simulink model "p7_2"  (R2024b)
settings: Solver=VariableStepAuto  StartTime=0.0  StopTime=10.0  RelTol=1e-3
libraries: simulink x2
settings Model: Creator=rouna  LastModifiedBy=rouna

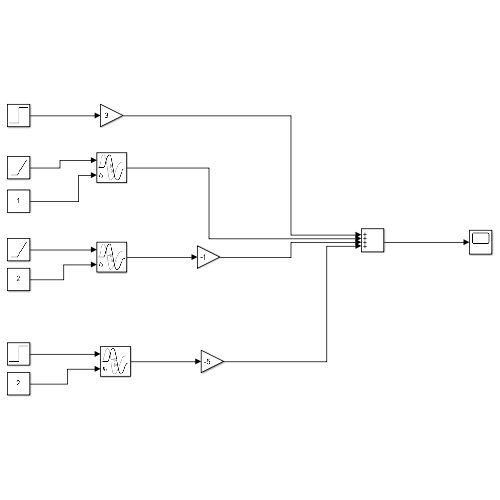
[thumbnail: Simulink's stored preview of the top-level diagram]
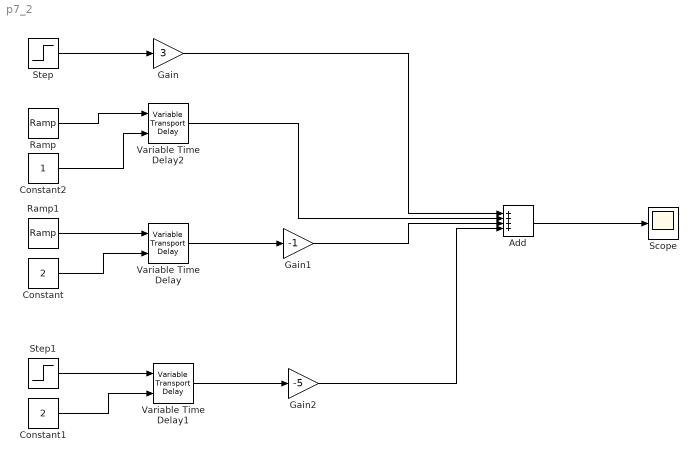
== system p7_2 ==
  Add : Sum  Inputs=++++
  Constant : Constant  Value=2
  Constant1 : Constant  Value=2
  Constant2 : Constant
  Gain : Gain  Gain=3
  Gain1 : Gain  Gain=-1
  Gain2 : Gain  Gain=-5
  Ramp : simulink/Sources/Ramp  slope=1  start=0  InitialOutput=0
  Ramp1 : simulink/Sources/Ramp  slope=1  start=0  InitialOutput=0
  Scope : Scope
  Step : Step  SampleTime=0
  Step1 : Step  SampleTime=0
  Variable Time Delay : VariableTransportDelay  MaximumDelay=10
  Variable Time Delay1 : VariableTransportDelay  MaximumDelay=10
  Variable Time Delay2 : VariableTransportDelay  MaximumDelay=10
  wires:
  Step/1 -> Gain/1
  Ramp1/1 -> Variable Time Delay/1
  Constant/1 -> Variable Time Delay/2
  Variable Time Delay/1 -> Gain1/1
  Variable Time Delay1/1 -> Gain2/1
  Step1/1 -> Variable Time Delay1/1
  Constant1/1 -> Variable Time Delay1/2
  Gain/1 -> Add/1
  Gain1/1 -> Add/3
  Gain2/1 -> Add/4
  Add/1 -> Scope/1
  Ramp/1 -> Variable Time Delay2/1
  Constant2/1 -> Variable Time Delay2/2
  Variable Time Delay2/1 -> Add/2
